simulink model "SysIden_Plant"  (R2025b)
settings: Solver=FixedStepAuto  StartTime=0.0  StopTime=250  RelTol=1e-3  EnableMultiTasking=on
libraries: slident x2, SignalEditorBlockLib x1
settings Model: PacingRate=3  ExtModeTrigDuration=2  Creator=PattarapolSangaroon  LastModifiedBy=PattarapolSangaroon
settings SolverCC: AutoInsertRateTranBlk=on
settings DataIOCC: SaveOutput=off  SaveTime=off
settings OptimizationCC: EnhancedBackFolding=on  PassReuseOutputArgsAs=Individual arguments  ZeroExternalMemoryAtStartup=off  ZeroInternalMemoryAtStartup=off  MaxStackSize=64  OptimizeBlockOrder=speed  DifferentSizesBufferReuse=on  EfficientTunableParamExpr=on
settings DebuggingCC: ParameterTunabilityLossMsg=error
settings HardwareCC: ProdBitPerInt=16.0  ProdBitPerPointer=16.0  ProdBitPerSizeT=16.0  ProdBitPerPtrDiffT=16.0  ProdLargestAtomicFloat=None  ProdWordSize=8.0  ProdHWDeviceType=Atmel->AVR
settings SFSimCC: MATLABDynamicMemAlloc=off
settings RTWCC: SystemTargetFile=ert.tlc  HardwareBoard=Arduino Uno  TemplateMakefile=ert_default_tmf  GenerateReport=on  Toolchain=Arduino AVR  BuildConfiguration=Faster Runs  Description=Embedded Coder
settings CodeAppCC: ForceParamTrailComments=on  IgnoreCustomStorageClasses=off  OperatorAnnotations=on  SimulinkDataObjDesc=on  SFDataObjDesc=on  InsertBlockDesc=on
settings ERTTargetCC: ExtModeTransport=3.0  ExtModeStaticAlloc=on  ExtModeAutomaticAllocSize=off  ExtModeStaticAllocSize=250.0  ExtModeMexFile=ext_xcp  ExtModeIntrfLevel=Level2 - Open  InlinedParameterPlacement=Hierarchical  SupportContinuousTime=on  SupportVariableSizeSignals=on

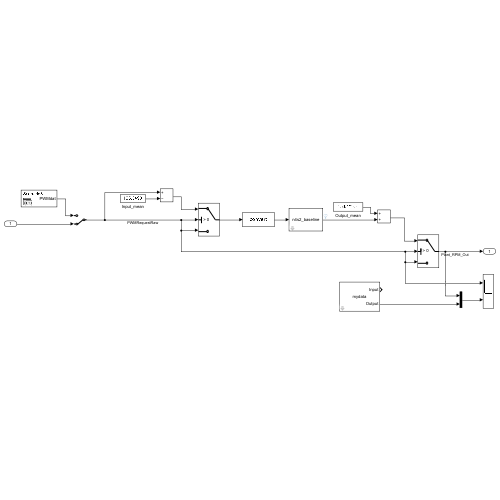
[thumbnail: Simulink's stored preview of the top-level diagram]
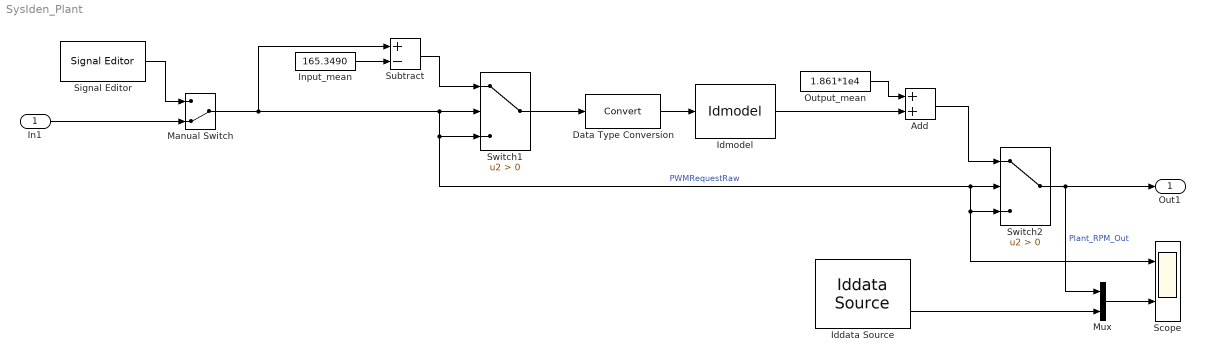
== system SysIden_Plant ==
  In1 : Inport  OutDataTypeStr=double  PortDimensions=1  SampleTime=0
  Add : Sum
  Data Type Conversion : DataTypeConversion  SaturateOnIntegerOverflow=off  RndMeth=Floor
  Iddata Source : slident/Iddata Source  iddataobj=mydata  T0=-1
  Idmodel : slident/Models/Idmodel  sys=n4s2_baseline  IC=0  noi=off  seed=[]
  Input_mean : Constant  Value=165.3490
  Manual Switch : ManualSwitch  CurrentSetting=0
  Mux : Mux  Inputs=2
  Output_mean : Constant  Value=1.861*1e4
  Scope : Scope  NumInputPorts=2
      settings: ActiveDisplayYMinimum=-29.999999999999993  ActiveDisplayYMaximum=270
  Signal Editor : SignalEditorBlockLib/Signal Editor  FileName=Signal_Editor_PWM_Sweep_0_255.mat  ActiveScenario=Scenario3  ActiveSignal=PWMdat  IsBus=off  OutputBusObjectStr=Bus: BusObject  SampleTime=0  Interpolate=off  ZeroCross=off  OutputAfterFinalValue=Setting to zero  Unit=inherit  PreserveSignalName=on  ApplySigPropsToAllScenarios=on  ApplySigPropsToAllSignals=off  SignalPropertySource=Dialog parameters
  Subtract : Sum  Inputs=+-
  Switch1 : Switch  Criteria=u2 > Threshold  SaturateOnIntegerOverflow=off  InputSameDT=off
  Switch2 : Switch  Criteria=u2 > Threshold  SaturateOnIntegerOverflow=off  InputSameDT=off
  Out1 : Outport  OutDataTypeStr=double  PortDimensions=1  SampleTime=0
  wires:
  Manual Switch/1 -> Switch1/2, Switch1/3, Scope/1, Switch2/3, Switch2/2, Subtract/1  "PWMRequestRaw"
  Subtract/1 -> Switch1/1
  Input_mean/1 -> Subtract/2
  Switch1/1 -> Data Type Conversion/1
  Switch2/1 -> Out1/1, Mux/1  "Plant_RPM_Out"
  Data Type Conversion/1 -> Idmodel/1
  Idmodel/1 -> Add/2
  Output_mean/1 -> Add/1
  Add/1 -> Switch2/1
  Mux/1 -> Scope/2
  Iddata Source/2 -> Mux/2
  In1/1 -> Manual Switch/2
  Signal Editor/1 -> Manual Switch/1
